simulink model "hyd_hyb_2_fuz_5cyc"  (Simulink 7.7)
settings: Solver=ode14x  StartTime=0  StopTime=12390  FixedStep=0.01  MaxStep=.4  RelTol=1e-8
InitFcn:
  | const_3
values from neighbouring files (symbols this model uses):
  Af = 6.3    [brk_enrg.m]    (also in brk_enrg_1.m)
  BSFC_906_205 = [3.5684 4.3466 5.1668 6.0769 6.988 7.8992 8.8104 9.7336 10.8548 11.9809 13.1112 14.2571 ... (663 elements, 39x17)]    [BSFC_map_906_205.mat]
  Cd = 0.55    [brk_enrg.m]    (also in brk_enrg_1.m)
  den = 1.202    [brk_enrg.m]    (also in brk_enrg_1.m)
  fr = 0.01    [brk_enrg.m]    (also in brk_enrg_1.m)
undefined symbols (not defined in the file or in its folder): clutchRise, down_spd_2, down_spd_3, down_spd_4, down_spd_c, fuel_density, gearshift, I_wheel, Idle_spd_eng_906, M1_hydr, p_v_15, pmax_125, qv_125, Rw, sec_eng_sfc_map, T_max_906, T_min, TC_spd_ratio_max, torque_convertor, Twait, up_spd_1, up_spd_2, up_spd_3, up_spd_c, v_p_10, v_p_15, v_p_5
libraries: fl_lib x43, nesl_utility x30, sdl_lib x14, simulink x4, fuzblock x1, simulink_need_slupdate x1
(part 1 of 2)
settings Model: Creator=Hybrid  LastModifiedBy=ali
settings SolverCC: MaxOrder=2  ZeroCrossControl=EnableAll
settings OptimizationCC: InitFltsAndDblsToZero=on
settings DebuggingCC: SaveWithParameterizedLinksMsg=none  SignalResolutionControl=TryResolveAllWithWarning  SolverPrmCheckMsg=none  MultiTaskDSMMsg=warning  MultiTaskCondExecSysMsg=none  UnconnectedInputMsg=none  UnconnectedOutputMsg=none  UnconnectedLineMsg=none  StrictBusMsg=Warning
settings SFSimCC: SimParseCustomCode=off
settings RTWCC: IncludeERTFirstTime=on
settings GRTTargetCC: TargetFcnLib=ansi_tfl_tmw.mat

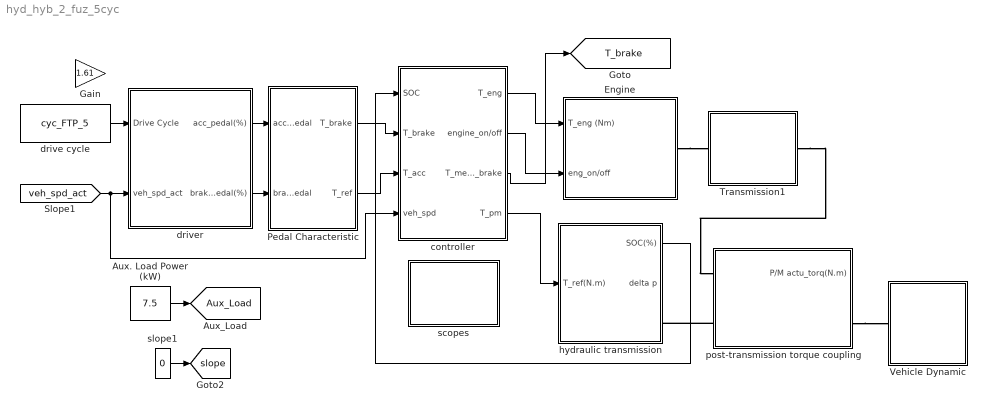
== system hyd_hyb_2_fuz_5cyc ==
  Aux. Load Power (kW) : Constant  Value=7.5
  Engine : Subsystem
  Gain : Gain  Gain=1.61
  Pedal Characteristic : Subsystem
  Transmission1 : Subsystem
  Vehicle Dynamic : Subsystem
  controller : Subsystem
  drive cycle : FromWorkspace  VariableName=cyc_FTP_5  SampleTime=0  OutputAfterFinalValue=Holding final value
  driver : Subsystem
      settings: MinAlgLoopOccurrences=on
  hydraulic transmission : Subsystem
  post-transmission torque coupling : Subsystem
  scopes : Subsystem
  slope1 : Constant  Value=0
  tag scope: Aux_Load=global, T_brake=global, slope=global
  wires:
  driver/2(brake_pedal(%)) -> Pedal Characteristic/2(brake_pedal)
  driver/1(acc_pedal(%)) -> Pedal Characteristic/1(acc_pedal)
  slope1/1 -> [slope]
  controller/1(T_eng) -> Engine/1(T_eng (Nm))
  controller/2(engine_on/off) -> Engine/2(eng_on/off)
  drive cycle/1 -> driver/1(Drive Cycle)
  [veh_spd_act] -> driver/2(veh_spd_act), controller/4(veh_spd)
  hydraulic transmission/1(SOC(%)) -> controller/1(SOC)
  Aux. Load Power (kW)/1 -> [Aux_Load]
  controller/3(T_mech_brake) -> [T_brake]
  controller/4(T_pm) -> hydraulic transmission/1(T_ref(N.m))
  Pedal Characteristic/2(T_ref) -> controller/3(T_acc)
  Pedal Characteristic/1(T_brake) -> controller/2(T_brake)
  connections:
  Engine/RConn1 -- Transmission1/LConn1
  post-transmission torque coupling/RConn1 -- Vehicle Dynamic/LConn1
  post-transmission torque coupling/LConn2 -- hydraulic transmission/RConn1
  Transmission1/RConn1 -- post-transmission torque coupling/LConn1

== system hyd_hyb_2_fuz_5cyc/Engine ==
  T_eng (Nm) : Inport
  eng_on/off : Inport  Port=2
  Consumption Calc (nmap)1 : Subsystem
  Engine Block : Subsystem
  Sensor(eng) : Subsystem
  eng_torq_estimator : Subsystem
  engine drag power : Subsystem
  idle speed control : Subsystem
  rasps2rpm : Gain  Gain=30/pi
  rasps2rpm1 : Gain  Gain=30/pi
  rasps2rpm2 : Gain  Gain=30/pi
  Transmission : PMIOPort  Port=1  Side=Right
  tag scope: T_out_idle_cotl=global, cons_LitP100km=global
  wires:
  Consumption Calc (nmap)1/1(cons lit/100km1) -> [cons_LitP100km]
  [Distance] -> Consumption Calc (nmap)1/2(distance)
  T_eng (Nm)/1 -> idle speed control/3(T_eng)
  idle speed control/1(T_eng + Idle) -> eng_torq_estimator/2(eng_trq_in), [T_out_idle_cotl]
  eng_torq_estimator/2(eng_trq_out (Nm)) -> Engine Block/1(eng_trq)
  engine drag power/1(drag torque ( Nm)) -> eng_torq_estimator/3(eng_drag_trq)
  eng_torq_estimator/1(eng_trq_out (Nm) to consump) -> Consumption Calc (nmap)1/4(T_eng)
  [w_eng] -> rasps2rpm/1
  rasps2rpm/1 -> Consumption Calc (nmap)1/1(w_eng (rpm))
  [w_eng] -> rasps2rpm1/1
  rasps2rpm1/1 -> eng_torq_estimator/1(eng_spd (rpm))
  [w_eng] -> rasps2rpm2/1
  rasps2rpm2/1 -> idle speed control/2(spd), engine drag power/1(eng_spd(rpm))
  [idle_control] -> Consumption Calc (nmap)1/5(acc pedal)
  eng_on/off/1 -> idle speed control/1(on), Consumption Calc (nmap)1/3(on/off)
  connections:
  Engine Block/RConn1 -- Sensor(eng)/LConn1
  Sensor(eng)/RConn1 -- Transmission/RConn1

== system hyd_hyb_2_fuz_5cyc/Pedal Characteristic ==
  acc_pedal : Inport
  brake_pedal : Inport  Port=2
  Constant1 : Constant  Value=.25
  Constant2 : Constant  Value=0
  Gain : Gain  Gain=13
  Scope : Scope  NumInputPorts=3
      settings: YMin=95~1258.75~-1  YMax=105~1391.25~1  SaveName=ScopeData9  MaxDataPoints=500
  convert T to acc. pedal : Gain  Gain=T_max_906/100
  convert T to brake pedal : Gain  Gain=-T_min/100
  retarder step one activation : Switch  Criteria=u2 > Threshold
  T_brake : Outport
  T_ref : Outport  Port=2
  wires:
  acc_pedal/1 -> retarder step one activation/2, convert T to acc. pedal/1, Scope/1
  brake_pedal/1 -> convert T to brake pedal/1
  convert T to acc. pedal/1 -> Scope/2, T_ref/1
  Constant2/1 -> retarder step one activation/1
  Constant1/1 -> retarder step one activation/3
  convert T to brake pedal/1 -> Scope/3, Gain/1
  Gain/1 -> T_brake/1

== system hyd_hyb_2_fuz_5cyc/Transmission1 ==
  Gain : Gain  Gain=30/pi
  Sensor(GB_out) : Subsystem
  Sensor(TC_GB) : Subsystem
  T : Scope
      settings: YMin=-10  YMax=1000  SaveName=ScopeData8
  Torque Convertor : Subsystem
  gear box : Subsystem
  transmission control : Subsystem
  Engine : PMIOPort  Port=1  Side=Left
  Coupling : PMIOPort  Port=2  Side=Right
  tag scope: Clutch_num=global, Lockup_Clutch=global
  wires:
  [w_eng] -> Gain/1
  Torque Convertor/1(T) -> T/1
  Gain/1 -> transmission control/1(eng spd (rpm))
  transmission control/2(desired gear) -> [Clutch_num], gear box/1(control input (gear no.))
  transmission control/1(lock up cluch) -> [Lockup_Clutch], Torque Convertor/1(lock up cluch)
  connections:
  Torque Convertor/RConn1 -- Sensor(TC_GB)/LConn1
  Sensor(TC_GB)/RConn1 -- gear box/LConn1
  Torque Convertor/LConn1 -- Engine/RConn1
  gear box/RConn1 -- Sensor(GB_out)/LConn1
  Sensor(GB_out)/RConn1 -- Coupling/RConn1

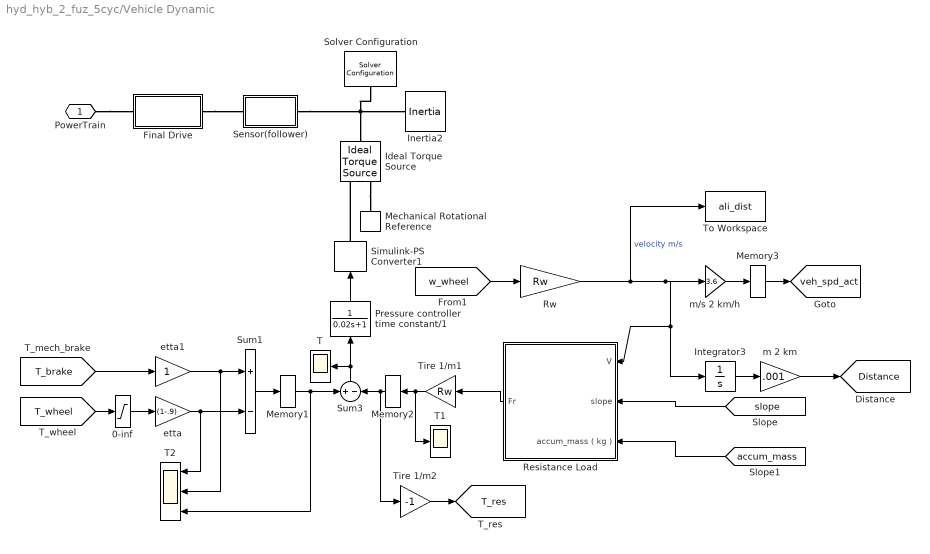
== system hyd_hyb_2_fuz_5cyc/Vehicle Dynamic ==
  0-inf : Saturate  UpperLimit=inf  LowerLimit=eps
  Final Drive : Subsystem
  Ideal Torque Source : fl_lib/Mechanical/Mechanical Sources/Ideal Torque Source  SystemSampleTime=-1  w_Log=off  t_Log=off  LocalVarNames=|w|t  LocalVarDescs=|w|t  LocalVarLogging=[0 0]
  Inertia2 : fl_lib/Mechanical/Rotational Elements/Inertia  SystemSampleTime=-1  inertia=I_wheel+M1_hydr*Rw^2 kg*m^2  initial_velocity=0 rad/s  t_Log=off  LocalVarNames=|t  LocalVarDescs=|t  LocalVarLogging=0
  Integrator3 : Integrator
  Mechanical Rotational Reference : fl_lib/Mechanical/Rotational Elements/Mechanical Rotational Reference  SystemSampleTime=-1  t_Log=off  LocalVarNames=|t  LocalVarDescs=|t  LocalVarLogging=0
  Memory1 : Memory
  Memory2 : Memory
  Memory3 : Memory
  Pressure controller time constant/1 : TransferFcn  Denominator=[0.02 1]
  Resistance Load : Subsystem
  Rw : Gain  Gain=Rw  SaturateOnIntegerOverflow=on  OutDataTypeStr=Inherit: Same as input  ParamDataTypeStr=Inherit: Same as input
  Sensor(follower) : Subsystem
  Simulink-PS Converter1 : nesl_utility/Simulink-PS Converter  SystemSampleTime=-1  PhysicalDomain=network_engine_domain  LeftPortType=input  RightPortType=output  SubClassName=ps_input  Unit=N*m  AffineConversion=off  InputFilterTimeConstant=0.01  UdotUserProvided=0
  Solver Configuration : nesl_utility/Solver Configuration  SystemSampleTime=-1  PhysicalDomain=network_engine_domain  LeftPortType=input  RightPortType=generic  SubClassName=solver  Accelerate=off  Profile=off  ResidualTolerance=1e-9  MaxNonlinIter=5  MaxModeIter=2  DoFixedCost=on  UseLocalSampling=off  DoDC=on  LinearAlgebra=Sparse  LocalSolverSampleTime=.01  LocalSolverChoice=NE_BACKWARD_EULER_ADVANCER  UseLocalSolver=on
  Sum1 : Sum  Inputs=+-  SaturateOnIntegerOverflow=on  InputSameDT=on  OutDataTypeStr=Inherit: Same as first input
  Sum3 : Sum  Inputs=+-  SaturateOnIntegerOverflow=on  InputSameDT=on  OutDataTypeStr=Inherit: Same as first input
  T : Scope
      settings: YMin=-7500  YMax=500  SaveName=ScopeData4
  T1 : Scope
      settings: SaveName=ScopeData12
  T2 : Scope  NumInputPorts=3
      settings: YMin=-100~-1~-1400  YMax=1400~1~100  SaveName=ScopeData15
  Tire 1/m1 : Gain  Gain=Rw  SaturateOnIntegerOverflow=on  OutDataTypeStr=Inherit: Same as input  ParamDataTypeStr=Inherit: Same as input
  Tire 1/m2 : Gain  Gain=-1  SaturateOnIntegerOverflow=on  OutDataTypeStr=Inherit: Same as input  ParamDataTypeStr=Inherit: Same as input
  To Workspace : ToWorkspace  VariableName=ali_dist  SampleTime=-1  SaveFormat=Structure With Time
  etta : Gain  Gain=(1-.9)
  etta1 : Gain
  m 2 km : Gain  Gain=.001
  m/s 2 km/h : Gain  Gain=3.6
  PowerTrain : PMIOPort  Port=1  Side=Left
  tag scope: Distance=global, T_res=global, veh_spd_act=global
  wires:
  [w_wheel] -> Rw/1
  Sum3/1 -> T/1, Pressure controller time constant/1/1
  Integrator3/1 -> m 2 km/1
  m 2 km/1 -> [Distance]
  m/s 2 km/h/1 -> Memory3/1
  Tire 1/m1/1 -> T1/1, Memory2/1
  [T_brake] -> etta1/1
  Sum1/1 -> Memory1/1
  etta/1 -> Sum1/2, T2/1
  etta1/1 -> Sum1/1, T2/2
  Rw/1 -> To Workspace/1, m/s 2 km/h/1, Integrator3/1, Resistance Load/1(V)  "velocity m/s"
  Memory2/1 -> Tire 1/m2/1, Sum3/2
  [T_wheel] -> 0-inf/1
  0-inf/1 -> etta/1
  Pressure controller time constant/1/1 -> Simulink-PS Converter1/1
  Tire 1/m2/1 -> [T_res]
  Memory1/1 -> Sum3/1, T2/3
  Memory3/1 -> [veh_spd_act]
  Resistance Load/1(Fr) -> Tire 1/m1/1
  [slope] -> Resistance Load/2(slope)
  [accum_mass] -> Resistance Load/3(accum_mass ( kg ))
  connections:
  PowerTrain/RConn1 -- Final Drive/LConn1
  Final Drive/RConn1 -- Sensor(follower)/LConn1
  Ideal Torque Source/RConn2 -- Mechanical Rotational Reference/LConn1
  Simulink-PS Converter1/RConn1 -- Ideal Torque Source/RConn1
  Sensor(follower)/RConn1 -- Inertia2/LConn1 -- Ideal Torque Source/LConn1 -- Solver Configuration/RConn1

== system hyd_hyb_2_fuz_5cyc/controller ==
  SOC : Inport
  T_brake : Inport  Port=2
  T_acc : Inport  Port=3
  veh_spd : Inport  Port=4
  Abs : Abs
  Abs1 : Abs
  Fuzzy Logic  Controller : fuzblock/Fuzzy Logic  Controller  SystemSampleTime=-1  fis=fuzy_controller1
  MATLAB Function : Stateflow chart  TreatAsAtomicUnit=on
  Mux : Mux  Inputs=3
  Switch : Switch  Criteria=u2 > Threshold  Threshold=0.1
  Switch1 : Switch  Criteria=u2 > Threshold
  on1 : Constant  Value=0
  on2 : Constant
  T_eng : Outport
  engine_on/off : Outport  Port=2
  T_mech_brake : Outport  Port=3
  T_pm : Outport  Port=4
  wires:
  on2/1 -> engine_on/off/1
  Mux/1 -> Fuzzy Logic  Controller/1
  veh_spd/1 -> Mux/1
  SOC/1 -> Mux/2
  T_brake/1 -> Abs/1, MATLAB Function/2(T_brk), Switch/1
  T_acc/1 -> Switch/3
  MATLAB Function/1(T_eng) -> T_eng/1
  MATLAB Function/2(T_mech_brk) -> T_mech_brake/1
  Abs1/1 -> Switch1/2
  Fuzzy Logic  Controller/1 -> Switch1/1
  on1/1 -> Switch1/3
  Switch1/1 -> MATLAB Function/1(T_pm), T_pm/1
  Switch/1 -> Mux/3, Abs1/1, MATLAB Function/3(T_dem)
  Abs/1 -> Switch/2

== system hyd_hyb_2_fuz_5cyc/driver ==
  Drive Cycle : Inport
  veh_spd_act : Inport  Port=2
  0 to inf1 : Saturate  UpperLimit=inf  LowerLimit=0
  0 to inf2 : Saturate  UpperLimit=inf  LowerLimit=0
  Chart : Stateflow chart  TreatAsAtomicUnit=on
  Derivative : Derivative
  Driver : Subsystem
  Mux : Mux  Inputs=2
  Subsystem : Subsystem
  Sum : Sum  Inputs=|+-
  T : Scope
      settings: SaveName=ScopeData20
  error : Subsystem
  acc_pedal(%) : Outport
  brake_pedal(%) : Outport  Port=2
  tag scope: driver_speed=global, driver_torque=global, trans_state=global
  wires:
  Drive Cycle/1 -> 0 to inf1/1  "Drive Cycle"
  Driver/1(T_dem) -> Subsystem/1(T_dem), [driver_torque]  "T_dem"
  veh_spd_act/1 -> 0 to inf2/1  "veh_spd"
  Sum/1 -> Driver/1(Error), error/1(error)  "error"
  Subsystem/1(acc_pedal(%)) -> acc_pedal(%)/1
  Subsystem/2(brake_pedal(%)) -> brake_pedal(%)/1
  Derivative/1 -> error/2(acceleration)
  0 to inf2/1 -> Sum/2, Driver/2(V_spd), Mux/2, Chart/2(speed)
  0 to inf1/1 -> Sum/1, Mux/1, Derivative/1, Chart/1(cyc)
  Mux/1 -> [driver_speed]
  Chart/1(s) -> T/1, [trans_state]

== system hyd_hyb_2_fuz_5cyc/hydraulic transmission ==
  T_ref(N.m) : Inport
  Memory : Memory
  Memory2 : Memory
  Mux : Mux  Inputs=2
  "PM_hydraulic_machine " : Subsystem
  Sensor(PM) : Subsystem
  Sum : Sum  Inputs=|+-
  accumulator : Subsystem
  conjunction with wheels : Subsystem
  controller : Subsystem
  gain : Gain
  init_SOC ( %) : Constant  Value=70
  l/min to l/s : Gain  Gain=(1/60)
  v(lit) : Integrator  InitialConditionSource=external
  to coupling : PMIOPort  Tag=PMCPort  Port=1  Side=Right
  SOC(%) : Outport
  delta p : Outport  Port=2
  tag scope: SoC=global, accum_mass=global
  wires:
  controller/1(vg(cm^3/rev)) -> "PM_hydraulic_machine "/3(vg(cm^3/rev)), conjunction with wheels/1(vg)
  Memory2/1 -> Mux/2, Sum/2
  Sum/1 -> controller/1(T_error)
  l/min to l/s/1 -> v(lit)/1
  gain/1 -> Memory2/1
  T_ref(N.m)/1 -> Sum/1, Mux/1
  "PM_hydraulic_machine "/3(delta p) -> delta p/1
  "PM_hydraulic_machine "/2(qv (lit/min)) -> l/min to l/s/1
  init_SOC ( %)/1 -> accumulator/2(init_SOC(%))
  v(lit)/1 -> accumulator/1(accum_vol(lit))
  accumulator/4(accum_init_vol(lit)) -> v(lit)/2
  accumulator/1(accum_pres(bar)) -> "PM_hydraulic_machine "/1(p_accum)
  accumulator/3(SOC_min(%)) -> "PM_hydraulic_machine "/4(SOC_min(%))
  accumulator/2(SOC(%)) -> "PM_hydraulic_machine "/5(SOC), SOC(%)/1, [SoC]
  conjunction with wheels/2(torque feedback) -> gain/1
  conjunction with wheels/1(n ( rpm )) -> Memory/1
  "PM_hydraulic_machine "/1(T(N.m)) -> conjunction with wheels/2(T)
  Mux/1 -> ?
  accumulator/5(accum_mass ( kg )) -> [accum_mass]
  Memory/1 -> "PM_hydraulic_machine "/2(n(rpm))
  connections:
  Sensor(PM)/RConn1 -- to coupling/RConn1
  Sensor(PM)/LConn1 -- conjunction with wheels/RConn1

== system hyd_hyb_2_fuz_5cyc/post-transmission torque coupling ==
  Inertia : fl_lib/Mechanical/Rotational Elements/Inertia  SystemSampleTime=-1  inertia=8.5e-3 kg*m^2  initial_velocity=0 rad/s  t_Log=off  LocalVarNames=|t  LocalVarDescs=|t  LocalVarLogging=0
  Sensor(coupling) : Subsystem
  Simple Gear : sdl_lib/Gears/Simple Gear  SystemSampleTime=-1  ratio=1  rotation_direction=1  friction_model=1  T_noload=0.1 N*m  T_nom=5 N*m  efficiency_nom=0.8  efficiency=0.8  mu_visc=[ 0 0 ] N*m/(rad/s)  w_thr=0.01 rad/s  LocalVarLogging=[]
  Simple Gear1 : sdl_lib/Gears/Simple Gear  SystemSampleTime=-1  ratio=1  rotation_direction=1  friction_model=1  T_noload=0.1 N*m  T_nom=5 N*m  efficiency_nom=0.8  efficiency=0.8  mu_visc=[ 0 0 ] N*m/(rad/s)  w_thr=0.01 rad/s  LocalVarLogging=[]
  pm gearbox : Subsystem
  from engine : PMIOPort  Tag=PMCPort  Port=1  Side=Left
  from P/M : PMIOPort  Tag=PMCPort  Port=2  Side=Left
  to the wheel : PMIOPort  Tag=PMCPort  Port=3  Side=Right
  P/M actu_torq(N.m) : Outport
  wires:
  pm gearbox/1(P/M actu_torq(N.m)) -> P/M actu_torq(N.m)/1
  connections:
  Simple Gear/LConn1 -- from engine/RConn1
  from P/M/RConn1 -- pm gearbox/LConn1
  pm gearbox/RConn1 -- Simple Gear1/LConn1 -- Inertia/LConn1
  Sensor(coupling)/LConn1 -- Simple Gear/RConn1 -- Simple Gear1/RConn1
  to the wheel/RConn1 -- Sensor(coupling)/RConn1

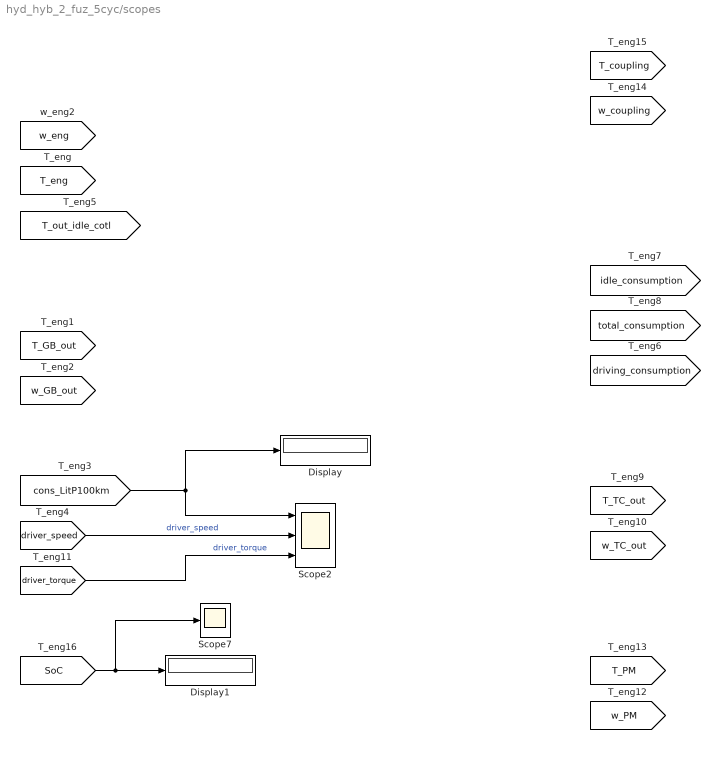
== system hyd_hyb_2_fuz_5cyc/scopes ==
  Display : Display
  Display1 : Display
  Scope2 : Scope  NumInputPorts=3
      settings: YMin=0~0~-1000  YMax=3e+016~45~1750  SaveName=driver_scope
  Scope7 : Scope
      settings: YMin=12  YMax=19  SaveName=gearbox_scope1
  wires:
  [cons_LitP100km] -> Scope2/1, Display/1
  [driver_speed] -> Scope2/2  "driver_speed"
  [driver_torque] -> Scope2/3  "driver_torque"
  [SoC] -> Display1/1, Scope7/1

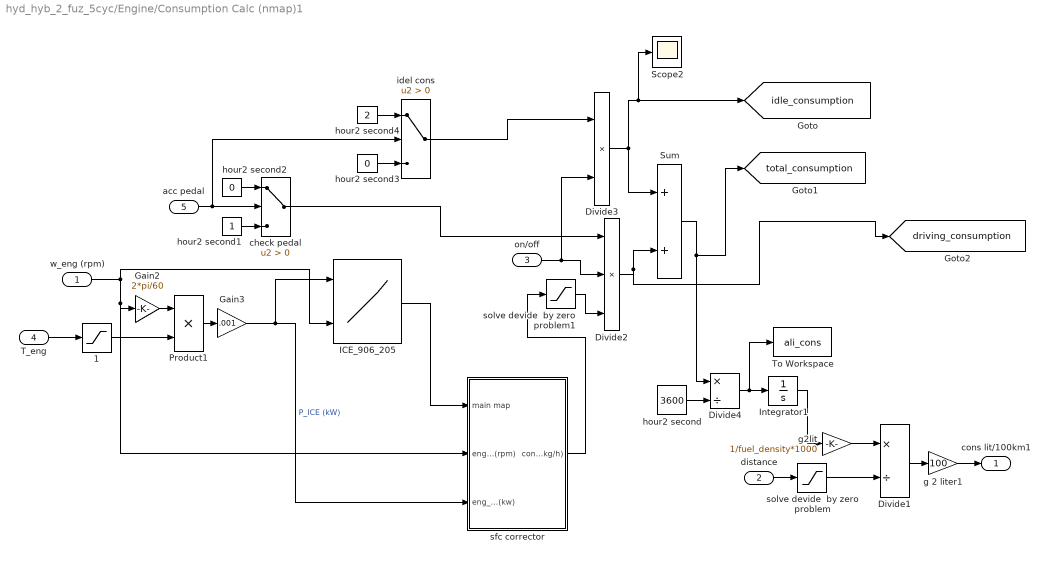
== system hyd_hyb_2_fuz_5cyc/Engine/Consumption Calc (nmap)1 ==
  w_eng (rpm) : Inport
  distance : Inport  Port=2
  on/off : Inport  Port=3
  T_eng : Inport  Port=4
  acc pedal : Inport  Port=5
  1 : Saturate  UpperLimit=inf  LowerLimit=0
  Divide1 : Product  Inputs=*/
  Divide2 : Product  Inputs=3
  Divide3 : Product
  Divide4 : Product  Inputs=*/
  Gain2 : Gain  Gain=2*pi/60
  Gain3 : Gain  Gain=.001
  ICE_906_205 : Lookup2D  RowIndex=p_906_205  ColumnIndex=w_906_205  Table=BSFC_906_205
  Integrator1 : Integrator
  Product1 : Product  RndMeth=Zero
  Scope2 : Scope
      settings: SaveName=ScopeData75
  Sum : Sum
  To Workspace : ToWorkspace  VariableName=ali_cons  SampleTime=-1  SaveFormat=Structure With Time
  check pedal : Switch  Criteria=u2 > Threshold
  g 2 liter1 : Gain  Gain=100
  g2lit : Gain  Gain=1/fuel_density*1000
  hour2 second : Constant  Value=3600
  hour2 second1 : Constant
  hour2 second2 : Constant  Value=0
  hour2 second3 : Constant  Value=0
  hour2 second4 : Constant  Value=2
  idel cons : Switch  Criteria=u2 > Threshold
  sfc corrector : Subsystem
  solve devide  by zero problem : Saturate  UpperLimit=inf  LowerLimit=eps
  solve devide  by zero problem1 : Saturate  UpperLimit=inf  LowerLimit=0
  cons lit/100km1 : Outport
  tag scope: driving_consumption=global, idle_consumption=global, total_consumption=global
  wires:
  Sum/1 -> Divide4/1, [total_consumption]
  1/1 -> Product1/2
  T_eng/1 -> 1/1
  w_eng (rpm)/1 -> Gain2/1, sfc corrector/2(eng_spd(rpm)), ICE_906_205/2
  hour2 second/1 -> Divide4/2
  Gain3/1 -> ICE_906_205/1, sfc corrector/3(eng_pow(kw))  "P_ICE (kW)"
  distance/1 -> solve devide  by zero problem/1
  solve devide  by zero problem/1 -> Divide1/2
  g 2 liter1/1 -> cons lit/100km1/1
  Divide1/1 -> g 2 liter1/1
  g2lit/1 -> Divide1/1
  Integrator1/1 -> g2lit/1
  Divide4/1 -> Integrator1/1, To Workspace/1
  Product1/1 -> Gain3/1
  Gain2/1 -> Product1/1
  sfc corrector/1(cons(kg/h)) -> solve devide  by zero problem1/1
  Divide2/1 -> Sum/2, [driving_consumption]
  hour2 second3/1 -> idel cons/3
  hour2 second4/1 -> idel cons/1
  solve devide  by zero problem1/1 -> Divide2/3
  on/off/1 -> Divide2/2, Divide3/2
  acc pedal/1 -> check pedal/2, idel cons/2
  hour2 second1/1 -> check pedal/3
  hour2 second2/1 -> check pedal/1
  check pedal/1 -> Divide2/1
  Divide3/1 -> Sum/1, [idle_consumption], Scope2/1
  idel cons/1 -> Divide3/1
  ICE_906_205/1 -> sfc corrector/1(main map)

== system hyd_hyb_2_fuz_5cyc/Engine/Engine Block ==
  eng_trq : Inport
  Ideal Torque Source : fl_lib/Mechanical/Mechanical Sources/Ideal Torque Source  SystemSampleTime=-1  w_Log=off  t_Log=off  LocalVarNames=|w|t  LocalVarDescs=|w|t  LocalVarLogging=[0 0]
  Inertia : fl_lib/Mechanical/Rotational Elements/Inertia  SystemSampleTime=-1  inertia=I_ICE kg*m^2  initial_velocity=0 rad/s  t_Log=off  LocalVarNames=|t  LocalVarDescs=|t  LocalVarLogging=0
  Mechanical Rotational Reference : fl_lib/Mechanical/Rotational Elements/Mechanical Rotational Reference  SystemSampleTime=-1  t_Log=off  LocalVarNames=|t  LocalVarDescs=|t  LocalVarLogging=0
  Memory : Memory  InheritSampleTime=on
  Simulink-PS Converter : nesl_utility/Simulink-PS Converter  SystemSampleTime=-1  PhysicalDomain=network_engine_domain  LeftPortType=input  RightPortType=output  SubClassName=ps_input  Unit=1  AffineConversion=off  InputFilterTimeConstant=0.01  UdotUserProvided=0
  Engine : PMIOPort  Port=1  Side=Right
  wires:
  eng_trq/1 -> Memory/1
  Memory/1 -> Simulink-PS Converter/1
  connections:
  Mechanical Rotational Reference/LConn1 -- Ideal Torque Source/RConn2
  Simulink-PS Converter/RConn1 -- Ideal Torque Source/RConn1
  Inertia/LConn1 -- Ideal Torque Source/LConn1 -- Engine/RConn1

== system hyd_hyb_2_fuz_5cyc/Engine/Sensor(eng) ==
  Motion sensor : Subsystem
  Torque sensor : Subsystem
  A : PMIOPort  Port=1  Side=Left
  B : PMIOPort  Port=2  Side=Right
  tag scope: T_eng=global, w_eng=global
  wires:
  Torque sensor/1(T) -> [T_eng]
  Motion sensor/1(W) -> [w_eng]
  connections:
  B/RConn1 -- Torque sensor/RConn1
  Torque sensor/LConn1 -- Motion sensor/LConn1 -- A/RConn1

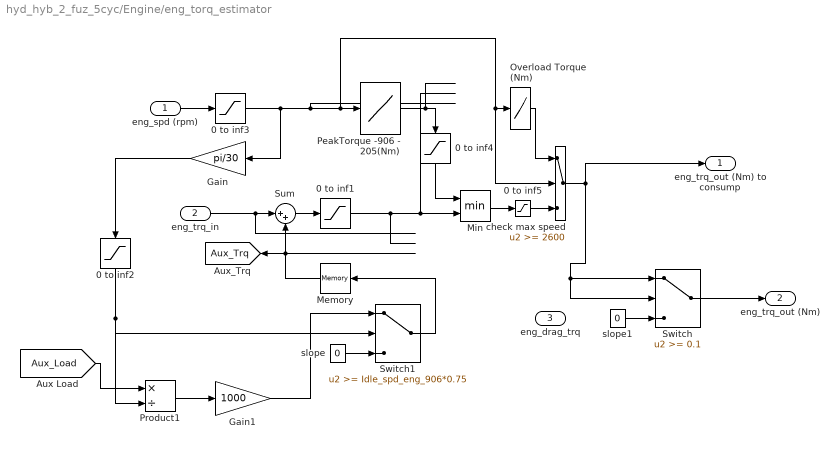
== system hyd_hyb_2_fuz_5cyc/Engine/eng_torq_estimator ==
  eng_spd (rpm) : Inport
  eng_trq_in : Inport  Port=2
  eng_drag_trq : Inport  Port=3
  0 to inf{1,3..5} (4 alike) : Saturate  UpperLimit=inf  LowerLimit=0
  0 to inf2 : Saturate  UpperLimit=inf  LowerLimit=eps
  Gain : Gain  Gain=pi/30
  Gain1 : Gain  Gain=1000
  Memory : Memory  InheritSampleTime=on
  Min : MinMax  Inputs=2
  Overload Torque (Nm) : Lookup  InputValues=[2600 2900 3000]  Table=[650 0 0]  SaturateOnIntegerOverflow=on
  PeakTorque -906 - 205(Nm) : Lookup  InputValues=[1000,1070,1130,1200,1280,1500,1590,1680,1760,1850,1930,2010,2070,2150,2240,2320,2380,2500]  Table=[982,1040,1080,1100,1110,1110,1100,1080,1060,1020,994,963,940,909,872,838,804,751]  SaturateOnIntegerOverflow=on
  Product1 : Product  Inputs=*/  RndMeth=Zero
  Sum : Sum  Inputs=|++
  Switch : Switch  Threshold=0.1
  Switch1 : Switch  Threshold=Idle_spd_eng_906*0.75
  check max speed : Switch  Threshold=2600
  slope : Constant  Value=0
  slope1 : Constant  Value=0
  eng_trq_out (Nm) to consump : Outport
  eng_trq_out (Nm) : Outport  Port=2
  tag scope: Aux_Trq=global
  wires:
  PeakTorque -906 - 205(Nm)/1 -> 0 to inf4/1
  check max speed/1 -> Switch/2, Switch/1, eng_trq_out (Nm) to consump/1
  0 to inf1/1 -> Min/2
  Overload Torque (Nm)/1 -> check max speed/1
  eng_spd (rpm)/1 -> 0 to inf3/1
  Switch/1 -> eng_trq_out (Nm)/1
  Gain/1 -> 0 to inf2/1
  eng_trq_in/1 -> Sum/1
  0 to inf2/1 -> Switch1/2, Product1/2
  Sum/1 -> 0 to inf1/1
  slope/1 -> Switch1/3
  Switch1/1 -> Memory/1
  Memory/1 -> Sum/2, [Aux_Trq]
  0 to inf3/1 -> Gain/1, Overload Torque (Nm)/1, check max speed/2, PeakTorque -906 - 205(Nm)/1
  0 to inf4/1 -> Min/1
  0 to inf5/1 -> check max speed/3
  Min/1 -> 0 to inf5/1
  [Aux_Load] -> Product1/1
  Product1/1 -> Gain1/1
  Gain1/1 -> Switch1/1
  slope1/1 -> Switch/3

== system hyd_hyb_2_fuz_5cyc/Engine/engine drag power ==
  eng_spd(rpm) : Inport
  0 to inf2 : Saturate  UpperLimit=inf  LowerLimit=eps
  Constant : Constant  Value=-1
  Gain : Gain  Gain=(pi)/30
  Gain1 : Gain  Gain=1000
  Scope : Scope  NumInputPorts=3
      settings: YMin=-5~-5~-5  YMax=5~5~5  SaveName=ScopeData2
  T_eng_drag (Nm) : Product  Inputs=/***
  engine_drag_power (kw) : Lookup  InputValues=[-10,eps,802.567507746791,824.568393094289,846.879150066401,868.8800354139,890.880920761399,912.881806108898,935.192563081009,957.193448428508,979.194333776007,1001.19521912351,1023.196104471,1045.1969898185,1067.197875166,1089.50863213811,1111.50951748561,1133.51040283311,1155.51128818061,1177.51217352811,1199.51305887561,1221.51394422311,1243.51482957061,1265.51571491811,1287.5166002656,1309.5174856131,1331.5183709606,1353.5192563081,1375.21027003099,1397.21115537849,1418.90216910137,1440.90305444887,1462.90393979637,1484.59495351926,1506.59583886676,1528.59672421425,1550.59760956175,1572.28862328464,1593.66976538291,1615.3607791058,1637.3616644533,1659.05267817618,1680.74369189907,1702.43470562196,1724.12571934484,1745.81673306773,1767.50774679062,1789.1987605135,1810.57990261178,1831.96104471005,1853.65205843294,1875.34307215582,1897.03408587871,1918.10535635237,1939.17662682603,1960.86764054892,1982.24878264719,2003.62992474546,2025.63081009296,2047.32182381585,2068.70296591412,2090.08410801239,3000]  Table=[0,0,8.89504100832017,9.50127747975726,9.88870415102495,10.2762179627945,10.7512208384311,11.1824791821341,11.6136503853353,12.0449087290384,12.4761670727414,12.9074254164445,13.294939228214,13.7261975719171,14.1137113836866,14.5448825868878,15.0636299944579,15.5386328700944,15.9698912137975,16.357405025567,16.7449188373366,17.1761771810396,17.6074355247427,17.9949493365122,18.4699522121488,18.9886996197188,19.4637024953554,20.026194434859,20.5887735148644,21.1950099863015,21.757589066307,22.2325919419435,22.7075948175801,23.2701738975855,23.8764103690226,24.4826468404597,25.0451387799633,25.7389514557692,26.5203403359441,27.21415301175,27.8641340151206,28.5579466909266,29.3392484305996,30.076805638339,30.858107378012,31.639409117685,32.420710857358,33.202012597031,34.1146350730063,35.0710020809152,35.9397928844552,36.7210946241282,37.5461408957346,38.4151059802784,39.3278155967556,40.1966064002956,41.0654843443374,41.8906177564458,42.6280878236834,43.4093895633564,44.2345229754647,45.1034009195066,45.1034009195066]
  no engine drag ( if we want ) : Constant
  drag torque ( Nm) : Outport
  wires:
  Gain/1 -> T_eng_drag (Nm)/1, Scope/2
  Constant/1 -> T_eng_drag (Nm)/3
  Gain1/1 -> T_eng_drag (Nm)/2, Scope/3
  0 to inf2/1 -> engine_drag_power (kw)/1, Gain/1
  engine_drag_power (kw)/1 -> Gain1/1
  T_eng_drag (Nm)/1 -> drag torque ( Nm)/1, Scope/1
  no engine drag ( if we want )/1 -> T_eng_drag (Nm)/4
  eng_spd(rpm)/1 -> 0 to inf2/1

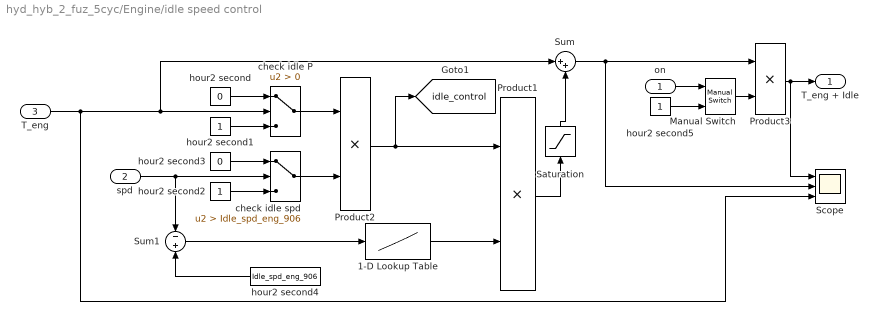
== system hyd_hyb_2_fuz_5cyc/Engine/idle speed control ==
  on : Inport
  spd : Inport  Port=2
  T_eng : Inport  Port=3
  1-D Lookup Table : Lookup_n-D  NumberOfTableDimensions=1  BreakpointsForDimension1=[0 Idle_spd_eng_906*0.025 Idle_spd_eng_906]  Table=[0 0 T_max_906/2]  RndMeth=Simplest  InputSameDT=on
  Manual Switch : simulink/Signal Routing/Manual Switch  SystemSampleTime=-1  sw=1  action=0  varsize=off
  Product1 : Product  Inputs=**  RndMeth=Zero
  Product2 : Product  Inputs=**  RndMeth=Zero
  Product3 : Product  Inputs=**  RndMeth=Zero
  Saturation : Saturate  UpperLimit=T_max_906/5  LowerLimit=0
  Scope : Scope  NumInputPorts=3
      settings: YMin=-5~-5~-5  YMax=5~5~5  SaveName=ScopeData11
  Sum : Sum  Inputs=|++
  Sum1 : Sum  Inputs=-|+
  check idle P : Switch  Criteria=u2 > Threshold
  check idle spd : Switch  Criteria=u2 > Threshold  Threshold=Idle_spd_eng_906
  hour2 second : Constant  Value=0
  hour2 second1 : Constant
  hour2 second2 : Constant
  hour2 second3 : Constant  Value=0
  hour2 second4 : Constant  Value=Idle_spd_eng_906
  hour2 second5 : Constant
  T_eng + Idle : Outport
  tag scope: idle_control=global
  wires:
  hour2 second4/1 -> Sum1/2
  Product1/1 -> Saturation/1
  Product2/1 -> Product1/1, [idle_control]
  Sum1/1 -> 1-D Lookup Table/1
  1-D Lookup Table/1 -> Product1/2
  check idle spd/1 -> Product2/2
  check idle P/1 -> Product2/1
  hour2 second2/1 -> check idle spd/3
  hour2 second3/1 -> check idle spd/1
  spd/1 -> Sum1/1, check idle spd/2
  hour2 second1/1 -> check idle P/3
  hour2 second/1 -> check idle P/1
  T_eng/1 -> check idle P/2, Sum/1, Scope/3
  Sum/1 -> Product3/1, Scope/2
  Product3/1 -> T_eng + Idle/1, Scope/1
  Manual Switch/1 -> Product3/2
  on/1 -> Manual Switch/1
  hour2 second5/1 -> Manual Switch/2
  Saturation/1 -> Sum/2

== system hyd_hyb_2_fuz_5cyc/Transmission1/Sensor(GB_out) ==
  Motion sensor : Subsystem
  Torque sensor : Subsystem
  A : PMIOPort  Port=1  Side=Left
  B : PMIOPort  Port=2  Side=Right
  tag scope: T_GB_out=global, w_GB_out=global
  wires:
  Motion sensor/1(W) -> [w_GB_out]
  Torque sensor/1(T) -> [T_GB_out]
  connections:
  A/RConn1 -- Motion sensor/LConn1 -- Torque sensor/LConn1
  B/RConn1 -- Torque sensor/RConn1

== system hyd_hyb_2_fuz_5cyc/Transmission1/Sensor(TC_GB) ==
  Motion sensor : Subsystem
  Torque sensor : Subsystem
  A : PMIOPort  Port=1  Side=Left
  B : PMIOPort  Port=2  Side=Right
  tag scope: T_TC_GB=global, w_TC_GB=global
  wires:
  Torque sensor/1(T) -> [T_TC_GB]
  Motion sensor/1(W) -> [w_TC_GB]
  connections:
  B/RConn1 -- Torque sensor/RConn1
  Torque sensor/LConn1 -- Motion sensor/LConn1 -- A/RConn1

== system hyd_hyb_2_fuz_5cyc/Transmission1/Torque Convertor ==
  note: Not: motoring mode is neglected
  lock up cluch : Inport
  " " : nesl_utility/Simulink-PS Converter  SystemSampleTime=-1  PhysicalDomain=network_engine_domain  LeftPortType=input  RightPortType=output  SubClassName=ps_input  Unit=1  AffineConversion=off  InputFilterTimeConstant=0.01  UdotUserProvided=0
  Clutch  Actuator : TransferFcn  Numerator=[1/clutchRise]  Denominator=[1 1/clutchRise]
  Disk Friction Clutch : sdl_lib/Clutches/Disk Friction Clutch  SystemSampleTime=-1  geometry_model=1  r_eff=1 m  d_o=150 mm  d_i=100 mm  nS=8  piston_area=0.001 m^2  friction_model=1  mu_coulomb=0.3  mu_w_vector=[ 0 0.1 0.2 0.3 0.4 0.5 1 2 5 10 100 1000 ] rad/s  mu_coulomb_vector=[ 0.29 0.28 0.26 0.22 0.21 0.2 0.2 0.19 0.19 0.19 0.19 0.19 ]  mu_interp_method=1  mu_extrap_method=1  mu_static=0.35  d_f=1  w_tol=0.001 rad/s  pressure_min=100 Pa  mu_visc=0 N*m/(rad/s)  initial_state_locked=0  LocalVarLogging=[]
  Gain : Gain  Gain=10e6
  Inertia : fl_lib/Mechanical/Rotational Elements/Inertia  SystemSampleTime=-1  inertia=Impeller_Inertia kg*m^2  initial_velocity=0 rad/s  t_Log=off  LocalVarNames=|t  LocalVarDescs=|t  LocalVarLogging=0
  Inertia1 : fl_lib/Mechanical/Rotational Elements/Inertia  SystemSampleTime=-1  inertia=Turbine_Inertia kg*m^2  initial_velocity=0 rad/s  t_Log=off  LocalVarNames=|t  LocalVarDescs=|t  LocalVarLogging=0
  main solver : Subsystem
  Impeller : PMIOPort  Port=1  Side=Left
  Turbine : PMIOPort  Port=2  Side=Right
  T : Outport
  wires:
  main solver/1(Turbine torque) -> T/1
  lock up cluch/1 -> Clutch  Actuator/1
  Clutch  Actuator/1 -> Gain/1
  Gain/1 -> " "/1
  connections:
  Inertia/LConn1 -- main solver/LConn1 -- Disk Friction Clutch/LConn2 -- Impeller/RConn1
  main solver/RConn1 -- Inertia1/LConn1 -- Turbine/RConn1 -- Disk Friction Clutch/RConn1
  " "/RConn1 -- Disk Friction Clutch/LConn1

== system hyd_hyb_2_fuz_5cyc/Transmission1/gear box ==
  note: Not: gear shift delay is not considered
  control input (gear no.) : Inport
  " " : nesl_utility/Simulink-PS Converter  SystemSampleTime=-1  PhysicalDomain=network_engine_domain  LeftPortType=input  RightPortType=output  SubClassName=ps_input  Unit=1  AffineConversion=off  InputFilterTimeConstant=0.01  UdotUserProvided=0
  1-D Lookup Table : Lookup_n-D  NumberOfTableDimensions=1  BreakpointsForDimension1=[-1 0 1 20]  Table=[0 0 1 1]  RndMeth=Simplest  InputSameDT=on
  Clutch  Actuator : TransferFcn  Numerator=[1/clutchRise]  Denominator=[1 1/clutchRise]
  Constant : Constant
  Disk Friction Clutch : sdl_lib/Clutches/Disk Friction Clutch  SystemSampleTime=-1  geometry_model=1  r_eff=1 m  d_o=150 mm  d_i=100 mm  nS=8  piston_area=0.001 m^2  friction_model=1  mu_coulomb=0.3  mu_w_vector=[ 0 0.1 0.2 0.3 0.4 0.5 1 2 5 10 100 1000 ] rad/s  mu_coulomb_vector=[ 0.29 0.28 0.26 0.22 0.21 0.2 0.2 0.19 0.19 0.19 0.19 0.19 ]  mu_interp_method=1  mu_extrap_method=1  mu_static=0.35  d_f=1  w_tol=0.001 rad/s  pressure_min=100 Pa  mu_visc=0 N*m/(rad/s)  initial_state_locked=0  LocalVarLogging=[]
  Gain : Gain  Gain=10e6
  Gain1 : Gain  Gain=Rw*3.6
  T : Scope
      settings: YMin=75  YMax=165  SaveName=ScopeData18
  gear box : Subsystem
  gear_inertia1 : fl_lib/Mechanical/Rotational Elements/Inertia  SystemSampleTime=-1  inertia=gear_inertia kg*m^2  initial_velocity=0 rad/s  t_Log=off  LocalVarNames=|t  LocalVarDescs=|t  LocalVarLogging=0
  gear_inertia2 : fl_lib/Mechanical/Rotational Elements/Inertia  SystemSampleTime=-1  inertia=gear_inertia kg*m^2  initial_velocity=0 rad/s  t_Log=off  LocalVarNames=|t  LocalVarDescs=|t  LocalVarLogging=0
  TC : PMIOPort  Port=1  Side=Left
  Coupling : PMIOPort  Port=2  Side=Right
  wires:
  control input (gear no.)/1 -> gear box/1(control signal)
  Gain/1 -> " "/1
  Clutch  Actuator/1 -> Gain/1
  [Drive_Cycle] -> Gain1/1
  Gain1/1 -> 1-D Lookup Table/1
  [trans_state] -> Clutch  Actuator/1, T/1
  connections:
  " "/RConn1 -- Disk Friction Clutch/LConn1
  Disk Friction Clutch/RConn1 -- Coupling/RConn1
  gear_inertia2/LConn1 -- Disk Friction Clutch/LConn2 -- gear box/RConn1
  gear box/LConn1 -- TC/RConn1 -- gear_inertia1/LConn1

== system hyd_hyb_2_fuz_5cyc/Transmission1/transmission control ==
  eng spd (rpm) : Inport
  Chart1 : Stateflow chart  TreatAsAtomicUnit=on
  control indictor1 : Scope
      settings: YMin=3.8  YMax=4.2  SaveName=ScopeData15
  engine speed : Scope
      settings: YMin=0  YMax=2200  SaveName=ScopeData32
  gear shift : MATLABFcn  MATLABFcn=gearshift(u(1))
  lock up cluch : Outport
  desired gear : Outport  Port=2
  wires:
  eng spd (rpm)/1 -> engine speed/1, Chart1/1(speed), gear shift/1
  Chart1/1(gear) -> desired gear/1
  Chart1/2(TC) -> lock up cluch/1
  gear shift/1 -> control indictor1/1

== system hyd_hyb_2_fuz_5cyc/Vehicle Dynamic/Final Drive ==
  Simple Gear : sdl_lib/Gears/Simple Gear  SystemSampleTime=-1  ratio=fd  rotation_direction=1  friction_model=1  T_noload=0.1 N*m  T_nom=5 N*m  efficiency_nom=0.8  efficiency=0.8  mu_visc=[ 0 0 ] N*m/(rad/s)  w_thr=0.01 rad/s  LocalVarLogging=[]
  engine : PMIOPort  Port=1  Side=Left
  Wheel : PMIOPort  Port=2  Side=Right
  connections:
  engine/RConn1 -- Simple Gear/LConn1
  Simple Gear/RConn1 -- Wheel/RConn1

== system hyd_hyb_2_fuz_5cyc/Vehicle Dynamic/Resistance Load ==
  note: Fg
  V : Inport
  slope : Inport  Port=2
  accum_mass ( kg ) : Inport  Port=3
  Aerodynamic Force : Subsystem
  Grade Force : Subsystem
  Rolling Force : Subsystem
  Sum1 : Sum  Inputs=+++  SaturateOnIntegerOverflow=on  InputSameDT=on  OutDataTypeStr=Inherit: Same as first input
  Fr : Outport
  wires:
  Grade Force/1(Fg) -> Sum1/3
  Aerodynamic Force/1(Fa) -> Sum1/1
  V/1 -> Aerodynamic Force/1(V), Rolling Force/1(V), Grade Force/2(V)
  Sum1/1 -> Fr/1
  slope/1 -> Grade Force/1(slope)
  Rolling Force/1(Fr) -> Sum1/2
  accum_mass ( kg )/1 -> Rolling Force/2(accum_mass), Grade Force/3(accum_mass)

== system hyd_hyb_2_fuz_5cyc/Vehicle Dynamic/Sensor(follower) ==
  Motion sensor : Subsystem
  Torque sensor : Subsystem
  A : PMIOPort  Port=1  Side=Left
  B : PMIOPort  Port=2  Side=Right
  tag scope: T_wheel=global, w_wheel=global
  wires:
  Torque sensor/1(T) -> [T_wheel]
  Motion sensor/1(W) -> [w_wheel]
  connections:
  B/RConn1 -- Torque sensor/RConn1
  Torque sensor/LConn1 -- Motion sensor/LConn1 -- A/RConn1

== system hyd_hyb_2_fuz_5cyc/driver/Driver ==
  Error : Inport
  V_spd : Inport  Port=2
  Derivative : Derivative
  Gain : Gain  Gain=100
  Gain1 : Gain  Gain=2
  Gain2 : Gain  Gain=0.5
  Gain3 : Gain  Gain=0
  Integrator : Integrator  ExternalReset=falling
  Scope : Scope  NumInputPorts=4
      settings: YMin=-1~-8000~-8000~-900  YMax=1~-5000~-5500~800  SaveName=ScopeData3
  Sum : Sum  Inputs=+++  RndMeth=Nearest  SaturateOnIntegerOverflow=on
  T_dem : Outport
  wires:
  Error/1 -> Gain/1
  Integrator/1 -> Gain2/1
  Sum/1 -> T_dem/1, Scope/2
  Gain/1 -> Integrator/1, Scope/4, Derivative/1, Gain1/1
  Gain2/1 -> Scope/3, Sum/3
  Derivative/1 -> Gain3/1
  Gain3/1 -> Sum/1, Scope/1
  V_spd/1 -> Integrator/2
  Gain1/1 -> Sum/2

== system hyd_hyb_2_fuz_5cyc/driver/Subsystem ==
  T_dem : Inport
  T_neg : Saturate  UpperLimit=0  LowerLimit=-100  ZeroCross=off
  T_pos : Saturate  UpperLimit=100  LowerLimit=0  ZeroCross=off
  convert T to acc. pedal : Gain  Gain=100/T_max_906
  convert T to brake pedal : Gain  Gain=100/T_min
  covert T to brake pedal1 : Gain  Gain=-1
  acc_pedal(%) : Outport
  brake_pedal(%) : Outport  Port=2
  wires:
  T_dem/1 -> convert T to acc. pedal/1, convert T to brake pedal/1
  convert T to acc. pedal/1 -> T_pos/1
  T_pos/1 -> acc_pedal(%)/1
  convert T to brake pedal/1 -> T_neg/1
  T_neg/1 -> covert T to brake pedal1/1
  covert T to brake pedal1/1 -> brake_pedal(%)/1

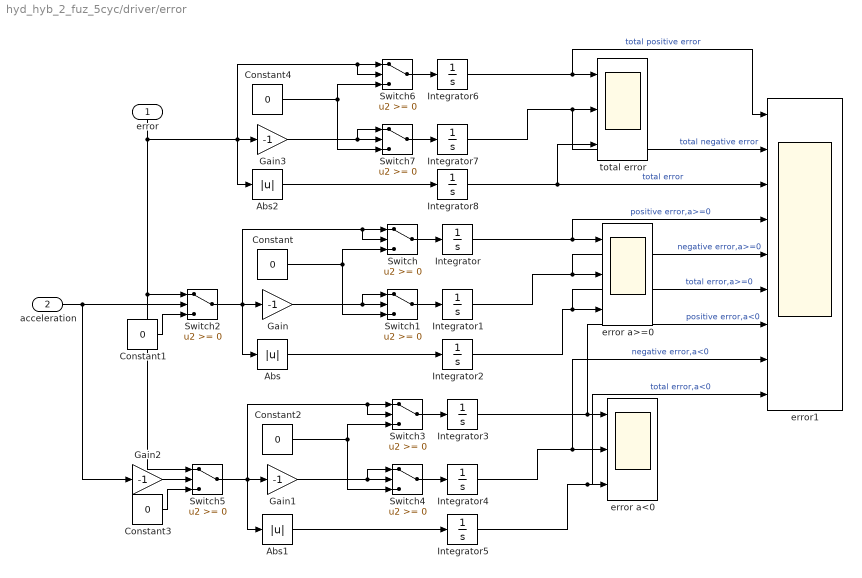
== system hyd_hyb_2_fuz_5cyc/driver/error ==
  error : Inport
  acceleration : Inport  Port=2
  Abs : Abs
  Abs1 : Abs
  Abs2 : Abs
  Constant{,1..4} (5 alike) : Constant  Value=0
  Gain{,1..3} (4 alike) : Gain  Gain=-1
  Integrator{,1..8} (9 alike) : Integrator
  Switch{,1..7} (8 alike) : Switch
  error a<0 : Scope  NumInputPorts=3
      settings: TimeRange=1800  YMin=51~12~62.5  YMax=73~15.25~90  SaveName=ScopeData14  MaxDataPoints=50000000
  error a>=0 : Scope  NumInputPorts=3
      settings: TimeRange=1800  YMin=0~0~0  YMax=2~6.5~8.5  SaveName=ScopeData13  MaxDataPoints=50000000
  error1 : Scope  NumInputPorts=9
      settings: TimeRange=1800  YMin=0~0~0~0~0~0~0~0~0  YMax=4~7.5~10~3~1~4~0.75~5~7.5  SaveName=ScopeData19  MaxDataPoints=50000000
  total error : Scope  NumInputPorts=3
      settings: TimeRange=1800  YMin=51~12~62.5  YMax=73~15.25~90  SaveName=ScopeData16  MaxDataPoints=50000000
  wires:
  Constant/1 -> Switch/3, Switch1/3
  Switch/1 -> Integrator/1
  Integrator/1 -> error a>=0/1, error1/4  "positive error,a>=0"
  Switch1/1 -> Integrator1/1
  Gain/1 -> Switch1/2, Switch1/1
  Integrator1/1 -> error a>=0/2, error1/5  "negative error,a>=0"
  Abs/1 -> Integrator2/1
  Integrator2/1 -> error a>=0/3, error1/6  "total error,a>=0"
  Switch2/1 -> Gain/1, Abs/1, Switch/1, Switch/2
  Constant1/1 -> Switch2/3
  Constant2/1 -> Switch4/3, Switch3/3
  Switch3/1 -> Integrator3/1
  Integrator3/1 -> error a<0/1, error1/7  "positive error,a<0"
  Switch4/1 -> Integrator4/1
  Gain1/1 -> Switch4/1, Switch4/2
  Integrator4/1 -> error a<0/2, error1/8  "negative error,a<0"
  Abs1/1 -> Integrator5/1
  Integrator5/1 -> error a<0/3, error1/9  "total error,a<0"
  Switch5/1 -> Switch3/2, Switch3/1, Abs1/1, Gain1/1
  Constant3/1 -> Switch5/3
  Gain2/1 -> Switch5/2
  Constant4/1 -> Switch7/3, Switch6/3
  Switch6/1 -> Integrator6/1
  Integrator6/1 -> total error/1, error1/1  "total positive error"
  Switch7/1 -> Integrator7/1
  Gain3/1 -> Switch7/1, Switch7/2
  Integrator7/1 -> total error/2, error1/2  "total negative error"
  Abs2/1 -> Integrator8/1
  Integrator8/1 -> total error/3, error1/3  "total error"
  error/1 -> Switch2/1, Switch5/1, Switch6/2, Switch6/1, Abs2/1, Gain3/1
  acceleration/1 -> Switch2/2, Gain2/1

== system hyd_hyb_2_fuz_5cyc/hydraulic transmission/PM_hydraulic_machine  ==
  p_accum : Inport
  n(rpm) : Inport  Port=2
  vg(cm^3/rev) : Inport  Port=3
  SOC_min(%) : Inport  Port=4
  SOC : Inport  Port=5
  Saturation1 : Saturate  UpperLimit=inf  LowerLimit=0.00001
  base variables : Subsystem
  eta estimator : Subsystem
  qv - pmax evaluation : Subsystem
  torque estimator : Subsystem
  T(N.m) : Outport
  qv (lit/min) : Outport  Port=2
  delta p : Outport  Port=3
  wires:
  qv - pmax evaluation/3(qv to etta) -> eta estimator/1(qv)
  qv - pmax evaluation/1(qv to accum) -> qv (lit/min)/1
  qv - pmax evaluation/2(pmax) -> eta estimator/3(Pmax)
  p_accum/1 -> base variables/1(p_accum)
  n(rpm)/1 -> base variables/2(n(rpm))
  vg(cm^3/rev)/1 -> base variables/3(vg(cm^3/rev))
  SOC_min(%)/1 -> base variables/4(SOC_min(%))
  SOC/1 -> base variables/5(SOC)
  base variables/1(vg) -> qv - pmax evaluation/5(vg), torque estimator/1(vg), eta estimator/4(vg)
  base variables/2(delta_p) -> qv - pmax evaluation/3(delta p), delta p/1, torque estimator/3(delta_p), eta estimator/2(delta_p)
  base variables/3(n) -> Saturation1/1, qv - pmax evaluation/4(n)
  base variables/4(SOC1) -> qv - pmax evaluation/1(SOC), torque estimator/5(SOC)
  base variables/5(SOC_min) -> qv - pmax evaluation/2(SOC_min(%))
  eta estimator/1(eta_mh) -> torque estimator/2(eta_mh)
  torque estimator/1(T(N.m)) -> T(N.m)/1
  Saturation1/1 -> eta estimator/5(n), torque estimator/4(n)
  qv - pmax evaluation/4(NAND - 1) -> torque estimator/6(NAND_1)
  torque estimator/2(NAND_2) -> qv - pmax evaluation/6(NAND - 2)

== system hyd_hyb_2_fuz_5cyc/hydraulic transmission/Sensor(PM) ==
  Motion sensor : Subsystem
  Torque sensor : Subsystem
  A : PMIOPort  Port=1  Side=Left
  B : PMIOPort  Port=2  Side=Right
  tag scope: T_PM=global, w_PM=global
  wires:
  Torque sensor/1(T) -> [T_PM]
  Motion sensor/1(W) -> [w_PM]
  connections:
  B/RConn1 -- Torque sensor/RConn1
  Torque sensor/LConn1 -- Motion sensor/LConn1 -- A/RConn1

== system hyd_hyb_2_fuz_5cyc/hydraulic transmission/accumulator ==
  accum_vol(lit) : Inport
  init_SOC(%) : Inport  Port=2
  SOC estimator : Subsystem
  accum_pres & vol estimator : Subsystem
  base variables : Subsystem
  max - min volume estimator : Subsystem
  accum_pres(bar) : Outport
  SOC(%) : Outport  Port=2
  SOC_min(%) : Outport  Port=3
  accum_init_vol(lit) : Outport  Port=4
  accum_mass ( kg ) : Outport  Port=5
  wires:
  accum_pres & vol estimator/1(accum_pres(bar)) -> accum_pres(bar)/1
  init_SOC(%)/1 -> base variables/1(init_SOC(%))
  accum_vol(lit)/1 -> base variables/2(accum_vol(lit))
  base variables/2(min_press) -> max - min volume estimator/1(min_press)
  base variables/3(max_press) -> max - min volume estimator/2(max_press)
  base variables/1(pre_ch_press) -> max - min volume estimator/3(pre_c_press), accum_pres & vol estimator/5(pre_ch_press(psi))
  base variables/4(accum_type) -> max - min volume estimator/4(accum_size), accum_pres & vol estimator/6(accum_type)
  accum_pres & vol estimator/2(accum_init_vol(lit)) -> accum_init_vol(lit)/1
  SOC estimator/1(SOC(%)) -> SOC(%)/1
  SOC estimator/2(SOC_min(%)) -> SOC_min(%)/1
  base variables/8(v_x) -> accum_pres & vol estimator/1(v_x), SOC estimator/2(v_x)
  max - min volume estimator/1(min_vol) -> SOC estimator/3(min_vol)
  base variables/5(accum_number) -> accum_pres & vol estimator/4(accum_num), max - min volume estimator/5(accum_num)
  base variables/6(init_SOC) -> accum_pres & vol estimator/2(init_SOC)
  max - min volume estimator/2(max_vol) -> accum_pres & vol estimator/3(max_vol), SOC estimator/1(max_vol)
  max - min volume estimator/3(accum_dry_mass ( kg )) -> accum_mass ( kg )/1

== system hyd_hyb_2_fuz_5cyc/hydraulic transmission/conjunction with wheels ==
  vg : Inport
  T : Inport  Port=2
  Constant : Constant  Value=0
  Ideal Rotational Motion Sensor : fl_lib/Mechanical/Mechanical Sensors/Ideal Rotational Motion Sensor  SystemSampleTime=-1  offset=0 rad  w_Log=off  t_Log=off  phi_Log=off  LocalVarNames=|w|t|phi  LocalVarDescs=|w|t|phi  LocalVarLogging=[0 0 0]
  Ideal Torque Source : fl_lib/Mechanical/Mechanical Sources/Ideal Torque Source  SystemSampleTime=-1  w_Log=off  t_Log=off  LocalVarNames=|w|t  LocalVarDescs=|w|t  LocalVarLogging=[0 0]
  Mechanical Rotational Reference : fl_lib/Mechanical/Rotational Elements/Mechanical Rotational Reference  SystemSampleTime=-1  t_Log=off  LocalVarNames=|t  LocalVarDescs=|t  LocalVarLogging=0
  Mechanical Rotational Reference1 : fl_lib/Mechanical/Rotational Elements/Mechanical Rotational Reference  SystemSampleTime=-1  t_Log=off  LocalVarNames=|t  LocalVarDescs=|t  LocalVarLogging=0
  PS-Simulink Converter : nesl_utility/PS-Simulink Converter  SystemSampleTime=-1  PhysicalDomain=network_engine_domain  LeftPortType=input  RightPortType=output  SubClassName=ps_output  Unit=1  AffineConversion=off
  Scope1 : Scope
      settings: YMin=-0.1  YMax=2  SaveName=ScopeData92
  Scope6 : Scope
      settings: YMin=-0.1  YMax=2  SaveName=ScopeData53
  Simulink-PS Converter : nesl_utility/Simulink-PS Converter  SystemSampleTime=-1  PhysicalDomain=network_engine_domain  LeftPortType=input  RightPortType=output  SubClassName=ps_input  Unit=1  AffineConversion=off  InputFilterTimeConstant=.001  UdotUserProvided=0
  Switch : Switch  Criteria=u2 ~= 0
  rad/s to rpm : Gain  Gain=60/(2*pi)
  Connection Port : PMIOPort  Tag=PMCPort  Port=1  Side=Right
  n ( rpm ) : Outport
  torque feedback : Outport  Port=2
  wires:
  Switch/1 -> torque feedback/1, Scope1/1, Simulink-PS Converter/1
  Constant/1 -> Switch/3
  vg/1 -> Switch/2
  PS-Simulink Converter/1 -> Scope6/1, rad/s to rpm/1
  rad/s to rpm/1 -> n ( rpm )/1
  T/1 -> Switch/1
  connections:
  Simulink-PS Converter/RConn1 -- Ideal Torque Source/RConn1
  Ideal Torque Source/RConn2 -- Mechanical Rotational Reference/LConn1
  Ideal Rotational Motion Sensor/LConn1 -- Connection Port/RConn1 -- Ideal Torque Source/LConn1
  Mechanical Rotational Reference1/LConn1 -- Ideal Rotational Motion Sensor/RConn1
  PS-Simulink Converter/LConn1 -- Ideal Rotational Motion Sensor/RConn2

== system hyd_hyb_2_fuz_5cyc/hydraulic transmission/controller ==
  T_error : Inport
  Gain : Gain  Gain=1.4
  PID Controller : simulink_need_slupdate/PID Controller  SystemSampleTime=-1  P=0.1  I=10  D=0
  Saturation : Saturate  UpperLimit=125  LowerLimit=-125
  Transfer Fcn : TransferFcn  Numerator=[1 0]  Denominator=[1 5]
  vg(cm^3/rev) : Outport
  wires:
  T_error/1 -> Gain/1
  Gain/1 -> PID Controller/1
  Saturation/1 -> vg(cm^3/rev)/1
  PID Controller/1 -> Transfer Fcn/1
  Transfer Fcn/1 -> Saturation/1

== system hyd_hyb_2_fuz_5cyc/post-transmission torque coupling/Sensor(coupling) ==
  Motion sensor : Subsystem
  Torque sensor : Subsystem
  A : PMIOPort  Port=1  Side=Left
  B : PMIOPort  Port=2  Side=Right
  tag scope: T_coupling=global, w_coupling=global
  wires:
  Torque sensor/1(T) -> [T_coupling]
  Motion sensor/1(W) -> [w_coupling]
  connections:
  B/RConn1 -- Torque sensor/RConn1
  Torque sensor/LConn1 -- Motion sensor/LConn1 -- A/RConn1

== system hyd_hyb_2_fuz_5cyc/post-transmission torque coupling/pm gearbox ==
  Ideal Torque Sensor : fl_lib/Mechanical/Mechanical Sensors/Ideal Torque Sensor  SystemSampleTime=-1  w_Log=off  t_Log=off  LocalVarNames=|w|t  LocalVarDescs=|w|t  LocalVarLogging=[0 0]
  Memory : Memory
  PS-Simulink Converter : nesl_utility/PS-Simulink Converter  SystemSampleTime=-1  PhysicalDomain=network_engine_domain  LeftPortType=input  RightPortType=output  SubClassName=ps_output  Unit=N*m  AffineConversion=off
  Simple Gear1 : sdl_lib/Gears/Simple Gear  SystemSampleTime=-1  ratio=1.75  rotation_direction=1  friction_model=1  T_noload=0.1 N*m  T_nom=5 N*m  efficiency_nom=0.8  efficiency=0.8  mu_visc=[ 0 0 ] N*m/(rad/s)  w_thr=0.01 rad/s  LocalVarLogging=[]
  Connection Port : PMIOPort  Tag=PMCPort  Port=1  Side=Left
  Connection Port1 : PMIOPort  Tag=PMCPort  Port=2  Side=Right
  P/M actu_torq(N.m) : Outport
  wires:
  Memory/1 -> P/M actu_torq(N.m)/1
  PS-Simulink Converter/1 -> Memory/1
  connections:
  Simple Gear1/LConn1 -- Connection Port/RConn1
  Simple Gear1/RConn1 -- Ideal Torque Sensor/LConn1
  Ideal Torque Sensor/RConn1 -- Connection Port1/RConn1
  Ideal Torque Sensor/RConn2 -- PS-Simulink Converter/LConn1

== system hyd_hyb_2_fuz_5cyc/Engine/Consumption Calc (nmap)1/sfc corrector ==
  main map : Inport
  eng_spd(rpm) : Inport  Port=2
  eng_pow(kw) : Inport  Port=3
  Constant : Constant  Value=Idle_spd_eng_906
  Constant1 : Constant  Value=1000
  Gain : Gain  Gain=-1
  Gain1 : Gain
  Gain2 : Gain
  Product : Product  Inputs=*/  RndMeth=Zero
  Product1 : Product  Inputs=*/  RndMeth=Zero
  Product2 : Product  RndMeth=Zero
  Product3 : Product  RndMeth=Zero
  Scope1 : Scope  NumInputPorts=2
      settings: YMin=-5~-5  YMax=5~5  SaveName=ScopeData41
  Scope2 : Scope  NumInputPorts=2
      settings: YMin=-5~-5  YMax=5~5  SaveName=ScopeData42
  Sum : Sum  Inputs=|+-
  Sum1 : Sum  Inputs=|+-
  Sum2 : Sum  Inputs=|+-
  Sum3 : Sum  Inputs=|++
  Switch : Switch  Threshold=1000
  sec_eng_sfc_map (906) : Lookup  InputValues=sec_eng_sfc_map(:,1)  Table=sec_eng_sfc_map(:,2)
  cons(kg/h) : Outport
  wires:
  Gain2/1 -> Product2/1, Scope2/2
  eng_pow(kw)/1 -> sec_eng_sfc_map (906)/1
  Switch/1 -> cons(kg/h)/1
  Sum3/1 -> Switch/3
  Product3/1 -> Sum3/2, Scope1/2
  Product2/1 -> Sum3/1, Scope1/1
  main map/1 -> Product3/1, Switch/1
  sec_eng_sfc_map (906)/1 -> Gain2/1, Scope2/1
  Product1/1 -> Product3/2  "b"
  Gain1/1 -> Product1/1
  Sum2/1 -> Gain1/1
  Product/1 -> Product2/2  "a"
  Sum1/1 -> Product1/2, Product/2
  Constant/1 -> Sum2/2, Sum1/2
  Gain/1 -> Product/1
  Sum/1 -> Gain/1
  Constant1/1 -> Sum1/1, Sum/2
  eng_spd(rpm)/1 -> Switch/2, Sum2/1, Sum/1

== system hyd_hyb_2_fuz_5cyc/Engine/Sensor(eng)/Motion sensor ==
  Ideal Rotational Motion Sensor : fl_lib/Mechanical/Mechanical Sensors/Ideal Rotational Motion Sensor  SystemSampleTime=-1  offset=0 rad  w_Log=off  t_Log=off  phi_Log=off  LocalVarNames=|w|t|phi  LocalVarDescs=|w|t|phi  LocalVarLogging=[]
  MRR : fl_lib/Mechanical/Rotational Elements/Mechanical Rotational Reference  SystemSampleTime=-1  t_Log=off  LocalVarNames=|t  LocalVarDescs=|t  LocalVarLogging=[]
  PS-Simulink Converter : nesl_utility/PS-Simulink Converter  SystemSampleTime=-1  PhysicalDomain=network_engine_domain  LeftPortType=input  RightPortType=output  SubClassName=ps_output  Unit=rad/s  AffineConversion=off
  A : PMIOPort  Port=1  Side=Left
  W : Outport
  wires:
  PS-Simulink Converter/1 -> W/1
  connections:
  MRR/LConn1 -- Ideal Rotational Motion Sensor/RConn1
  Ideal Rotational Motion Sensor/RConn2 -- PS-Simulink Converter/LConn1
  A/RConn1 -- Ideal Rotational Motion Sensor/LConn1

== system hyd_hyb_2_fuz_5cyc/Engine/Sensor(eng)/Torque sensor ==
  PS2S : nesl_utility/PS-Simulink Converter  SystemSampleTime=-1  PhysicalDomain=network_engine_domain  LeftPortType=input  RightPortType=output  SubClassName=ps_output  Unit=1  AffineConversion=off
  Torque Sensor : fl_lib/Mechanical/Mechanical Sensors/Ideal Torque Sensor  SystemSampleTime=-1  w_Log=off  t_Log=off  LocalVarNames=|w|t  LocalVarDescs=|w|t  LocalVarLogging=[]
  B : PMIOPort  Port=1  Side=Right
  A : PMIOPort  Port=2  Side=Left
  T : Outport
  wires:
  PS2S/1 -> T/1
  connections:
  Torque Sensor/RConn2 -- PS2S/LConn1
  B/RConn1 -- Torque Sensor/RConn1
  A/RConn1 -- Torque Sensor/LConn1

== system hyd_hyb_2_fuz_5cyc/Transmission1/Sensor(GB_out)/Motion sensor ==
  Ideal Rotational Motion Sensor : fl_lib/Mechanical/Mechanical Sensors/Ideal Rotational Motion Sensor  SystemSampleTime=-1  offset=0 rad  w_Log=off  t_Log=off  phi_Log=off  LocalVarNames=|w|t|phi  LocalVarDescs=|w|t|phi  LocalVarLogging=[]
  MRR : fl_lib/Mechanical/Rotational Elements/Mechanical Rotational Reference  SystemSampleTime=-1  t_Log=off  LocalVarNames=|t  LocalVarDescs=|t  LocalVarLogging=[]
  PS-Simulink Converter : nesl_utility/PS-Simulink Converter  SystemSampleTime=-1  PhysicalDomain=network_engine_domain  LeftPortType=input  RightPortType=output  SubClassName=ps_output  Unit=rad/s  AffineConversion=off
  A : PMIOPort  Port=1  Side=Left
  W : Outport
  wires:
  PS-Simulink Converter/1 -> W/1
  connections:
  A/RConn1 -- Ideal Rotational Motion Sensor/LConn1
  Ideal Rotational Motion Sensor/RConn2 -- PS-Simulink Converter/LConn1
  MRR/LConn1 -- Ideal Rotational Motion Sensor/RConn1
